simulink model "Lab_Haptic_Template3"  (R2022a)
settings: Solver=FixedStepDiscrete  StartTime=0.0  StopTime=inf  FixedStep=0.002  RelTol=1e-3  EnableMultiTasking=on
settings Model: SimulationMode=external  ExtModeTrigDuration=2  Creator=Ken Noé  LastModifiedBy=19jelg
settings SolverCC: AlgebraicLoopSolver=TrustRegion
settings OptimizationCC: EnhancedBackFolding=on  PassReuseOutputArgsThreshold=0  MaxStackSize=64  OptimizeBlockOrder=speed  DifferentSizesBufferReuse=on  OptimizationCustomize=off
settings DebuggingCC: ParameterTunabilityLossMsg=error  UnconnectedInputMsg=warning  UnconnectedOutputMsg=warning  UnconnectedLineMsg=warning  SFMachineParentedDataDiag=warning
settings HardwareCC: ProdBitPerInt=16  ProdBitPerPointer=16  ProdBitPerSizeT=16  ProdBitPerPtrDiffT=16  ProdLargestAtomicFloat=None  ProdWordSize=8  ProdHWDeviceType=Atmel->AVR  UseEmbeddedCoderFeatures=off  UseSimulinkCoderFeatures=off
settings SFSimCC: MATLABDynamicMemAlloc=off  CustomCodeUndefinedFunction=UseInterfaceOnly
settings RTWCC: SystemTargetFile=ert.tlc  HardwareBoard=Arduino Uno  TemplateMakefile=ert_default_tmf  RTWVerbose=off  Toolchain=Arduino AVR  BuildConfiguration=Faster Runs
settings CodeAppCC: ForceParamTrailComments=on  OperatorAnnotations=on  MangleLength=10
settings ERTTargetCC: ERTCustomFileBanners=off  SupportContinuousTime=on  SupportNonInlinedSFcns=on  RemoveResetFunc=off  SupportVariableSizeSignals=on  ModelStepFunctionPrototypeControlCompliant=off  ExtMode=on  ExtModeStaticAllocSize=250  ExtModeMexArgs='127.0.0.1' 0 17725  ERTSrcFileBannerTemplate=codertarget_code_template.cgt  ERTHdrFileBannerTemplate=codertarget_code_template.cgt  ERTDataSrcFileTemplate=codertarget_code_template.cgt  ERTDataHdrFileTemplate=codertarget_code_template.cgt

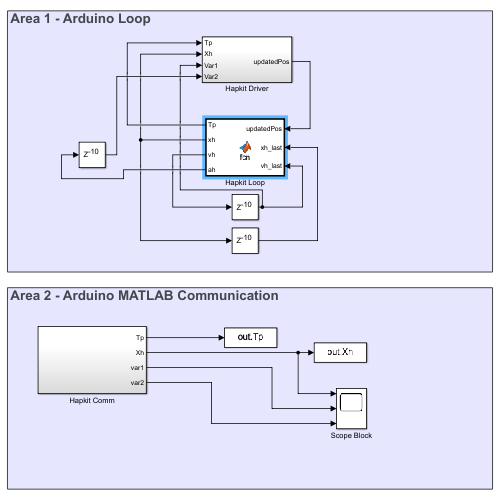
[thumbnail: Simulink's stored preview of the top-level diagram]
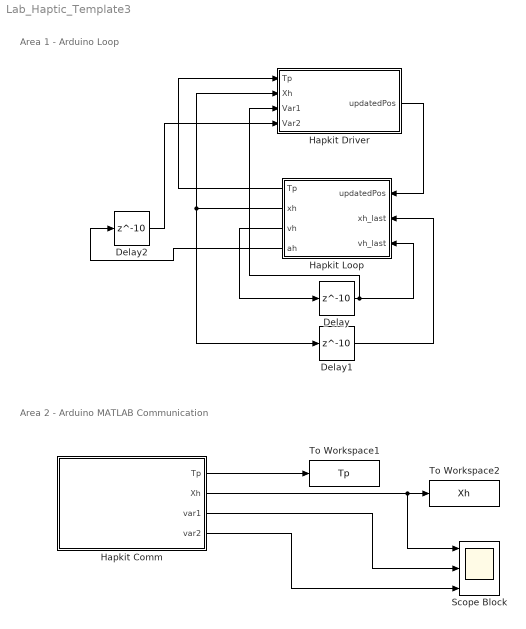
== system Lab_Haptic_Template3 ==
  note: Area 1 - Arduino Loop
  note: Area 2 - Arduino MATLAB Communication
  Delay : Delay  DelayLength=10
  Delay1 : Delay  DelayLength=10
  Delay2 : Delay  DelayLength=10
  Hapkit Comm : Subsystem
  Hapkit Driver : Subsystem
  Hapkit Loop : MATLAB Function  TreatAsAtomicUnit=on
  Scope Block : Scope  NumInputPorts=3
  To Workspace1 : ToWorkspace  VariableName=Tp  SampleTime=-1
      settings: Save2DSignal=2-D array (concatenate along first dimension)
  To Workspace2 : ToWorkspace  VariableName=Xh  SampleTime=-1
      settings: Save2DSignal=2-D array (concatenate along first dimension)
  wires:
  Hapkit Loop/3(vh) -> Delay/1
  Delay/1 -> Hapkit Driver/3(Var1), Hapkit Loop/3(vh_last)
  Hapkit Loop/1(Tp) -> Hapkit Driver/1(Tp)
  Hapkit Driver/1(updatedPos) -> Hapkit Loop/1(updatedPos)
  Hapkit Loop/2(xh) -> Delay1/1, Hapkit Driver/2(Xh)
  Delay1/1 -> Hapkit Loop/2(xh_last)
  Hapkit Comm/1(Tp) -> To Workspace1/1
  Hapkit Comm/2(Xh) -> Scope Block/1, To Workspace2/1
  Hapkit Comm/3(var1) -> Scope Block/2
  Hapkit Comm/4(var2) -> Scope Block/3
  Hapkit Loop/4(ah) -> Delay2/1
  Delay2/1 -> Hapkit Driver/4(Var2)

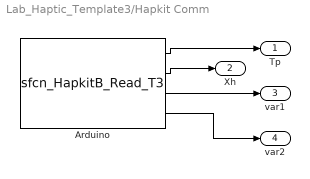
== system Lab_Haptic_Template3/Hapkit Comm ==
  Arduino : S-Function  InitFcn=try, set_param(gcb,'FunctionName','sfcn_HapkitB_Read_T3'), end  FunctionName=sfcn_HapkitB_Read_T3  SFunctionModules=sfcn_HapkitB_Read_T3_wrapper  SFunctionDeploymentMode=off  EnableBusSupport=off  mask(S-Function Builder){}
      mask help: Simulink:masks:SFunctionBuilder_MD
      mask init:
      | val = [[.9  0.75 0.75 1 1 .9 .9 1]',[1 1 0.75 0.75 .9 .9 1 .9]'];try , sys = get_param(gcb,'SfunBuilderFcnName');if isempty(sys), sys = get_param(gcb,'FunctionName'); end,catch, sys = get_param(gcb,'FunctionName'); end
      settings: CopyFcn=set_param(gcbh,'LinkStatus','none')  PreSaveFcn=try, set_param(gcb,'FunctionName','sfcn_HapkitB_Read_T3'), end  OpenFcn=sfunctionwizard(gcbh)
      mask Display:
      | plot(val(:,1),val(:,2))
      | disp(sys)
      | port_label('output',1,'Tp')
      | port_label('output',2,'Xh')
      | port_label('output',3,'var1')
      | port_label('output',4,'var2')
  Tp : Outport
  Xh : Outport  Port=2
  var1 : Outport  Port=3
  var2 : Outport  Port=4
  wires:
  Arduino/1 -> Tp/1
  Arduino/2 -> Xh/1
  Arduino/4 -> var2/1
  Arduino/3 -> var1/1

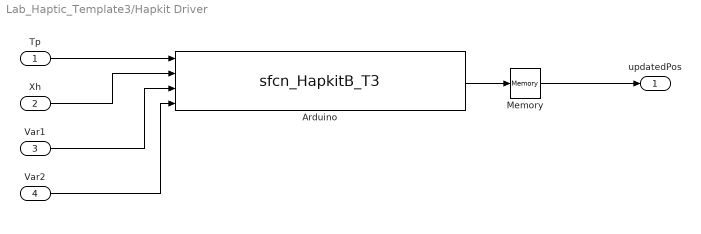
== system Lab_Haptic_Template3/Hapkit Driver ==
  Tp : Inport  OutDataTypeStr=single
  Xh : Inport  Port=2  OutDataTypeStr=single
  Var1 : Inport  Port=3  OutDataTypeStr=single
  Var2 : Inport  Port=4  OutDataTypeStr=single
  Arduino : S-Function  InitFcn=try, set_param(gcb,'FunctionName','sfcn_HapkitB_T3'), end  FunctionName=sfcn_HapkitB_T3  Parameters=uint8(uint8(2)),uint8(uint8(8)),uint8(uint8(5))  SFunctionModules=sfcn_HapkitB_T3_wrapper  SFunctionDeploymentMode=off  EnableBusSupport=off  mask(S-Function Builder){}
      mask help: Simulink:masks:SFunctionBuilder_MD
      mask init: same as Lab_Haptic_Template3/Hapkit Comm/Arduino
      settings: CopyFcn=set_param(gcbh,'LinkStatus','none')  PreSaveFcn=try, set_param(gcb,'FunctionName','sfcn_HapkitB_T3'), end  OpenFcn=sfunctionwizard(gcbh)
      mask Display:
      | plot(val(:,1),val(:,2))
      | disp(sys)
      | port_label('input',1,'Tp_in')
      | port_label('input',2,'Xh_in')
      | port_label('input',3,'var1_in')
      | port_label('input',4,'var2_in')
      | port_label('output',1,'updatedPos_out')
  Memory : Memory
  updatedPos : Outport
  wires:
  Tp/1 -> Arduino/1
  Arduino/1 -> Memory/1
  Memory/1 -> updatedPos/1
  Xh/1 -> Arduino/2
  Var1/1 -> Arduino/3
  Var2/1 -> Arduino/4

== matlab function Lab_Haptic_Template3/Hapkit Loop ==
  data: updatedPos input; Tp output single; xh_last input single; xh output single; vh_last input single; vh output single; ah output single
function [Tp,xh,vh,ah]  = fcn(updatedPos,xh_last,vh_last)
% function [outputs] = fcn(inputs)

%% Initialization
persistent t_discrete rp rh rs
if isempty(t_discrete)
    t_discrete = single(0); % Please do not change
    rp = 0.00575; % You set the rp value here
    rs = 0.073; % You set the rs value here
    rh = 0.089; % You set the rh value here
end

%% ****** Section 2. Compute position in meters *******************
ts = (-0.0128*updatedPos) +1.3253;
xh = 0.00579 * ts * 3.141592654/180;

%% Velocity estimation (vh)
vh  = (xh - xh_last) / 0.002;;
%% Acceleration estimation (ah)
ah  = (vh - vh_last) / 0.002;
%% Trajectory Generation

if (t_discrete < single(1)) % Wait one second to generate the sinewave
    t2 = single(0);
else
    t2 = single(t_discrete-1);
end

% trajectory = 0.025 * sin(2*pi*0.1 * t2); % Data1
% trajectory = 0.025 * sin(2*pi*0.1 * t2) + 0.007 * sin(2*pi*2.5 * t2); % Data2

%% PD controller
% force = 200 * (trajectory - xh) - 1 * vh ;

%% Virtual Environment
force = single(0);

%% Contact force estimation
% force_h_hat = single(0);

%% Force to Torque Mapping

Tp = force/172.7;
%% Discrete time (Please do not change)

t_discrete = t_discrete+0.002;
